simulink library "uavsimBlockset_Environment_turbulentWind"  (Simulink 8.6)
settings: Solver=ode45  StartTime=0.0  StopTime=10.0  RelTol=1e-3
undefined symbols (not defined in the file): F, Light, mask_ambientWind, mask_windON, mask_wingspan, MIL, uavsimblockset_cartesianToAngle
libraries: aerolibwind2 x1
settings Model: Creator=mstolle  LastModifiedBy=j.bolting

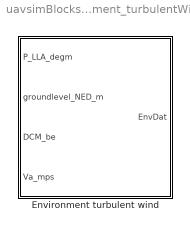
== system uavsimBlockset_Environment_turbulentWind ==
  Environment turbulent wind : Subsystem  mask{mask_constantwind_NED_mps=mask_ambientWind, mask_wingspan=mask_wingspan, mask_windON=mask_windON, mask_turbulenceON=1}
      mask prompts: mask_constantwind_NED_mps "Ambient, i.e. constant wind vector [m/s], NED frame"; mask_wingspan "Aircraft wingspan"; mask_windON "Ambient wind ON?"; mask_turbulenceON "Turbulence ON?"

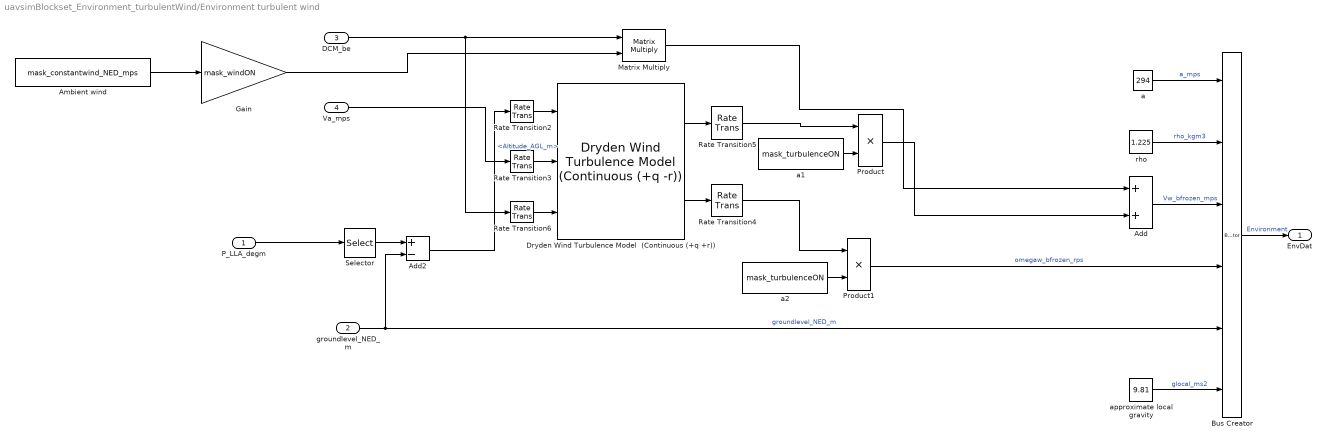
== system uavsimBlockset_Environment_turbulentWind/Environment turbulent wind ==
  P_LLA_degm : Inport
  groundlevel_NED_m : Inport  Port=2
  DCM_be : Inport  Port=3
  Va_mps : Inport  Port=4
  Add : Sum
  Add2 : Sum  Inputs=+-
  Ambient wind : Constant  Value=mask_constantwind_NED_mps
  Bus Creator : BusCreator  Inputs=6  OutDataTypeStr=Bus: Environment  NonVirtualBus=on
  Dryden Wind Turbulence Model  (Continuous (+q +r)) : aerolibwind2/Dryden Wind Turbulence Model  (Continuous (+q -r))  units=Metric (MKS)  spec=MIL-F-8785C  model=Discrete Dryden (+q -r)  W20=norm(mask_constantwind_NED_mps)  Wdeg=rad2deg(uavsimblockset_cartesianToAngle(mask_constantwind_NED_mps(1), mask_constantwind_NED_mps(2)))  TurbProb=10^-2 - Light  L_high=533.4  Wingspan=mask_wingspan  ts=0.1  Seed=randi(2^6, [1 4])  T_on=on
  Gain : Gain  Gain=mask_windON
  Matrix Multiply : Product  Multiplication=Matrix(*)
  Product : Product  RndMeth=Zero
  Product1 : Product  RndMeth=Zero
  Rate Transition2 : RateTransition  OutPortSampleTime=0.1
  Rate Transition3 : RateTransition  OutPortSampleTime=0.1
  Rate Transition4 : RateTransition  OutPortSampleTime=0
  Rate Transition5 : RateTransition  OutPortSampleTime=0
  Rate Transition6 : RateTransition  OutPortSampleTime=0.1
  Selector : Selector  InputPortWidth=3  IndexOptions=Index vector (dialog)  Indices=3  OutputSizes=1
  a : Constant  Value=294
  a1 : Constant  Value=mask_turbulenceON
  a2 : Constant  Value=mask_turbulenceON
  approximate local gravity : Constant  Value=9.81
  "rho " : Constant  Value=1.225
  EnvDat : Outport  OutDataTypeStr=Bus: Environment
  wires:
  Gain/1 -> Matrix Multiply/2
  Product1/1 -> Bus Creator/4  "omegaw_bfrozen_rps"
  a2/1 -> Product1/2
  a1/1 -> Product/2
  Product/1 -> Add/2
  Dryden Wind Turbulence Model  (Continuous (+q +r))/2 -> Rate Transition4/1
  P_LLA_degm/1 -> Selector/1
  groundlevel_NED_m/1 -> Add2/2, Bus Creator/5  "groundlevel_NED_m"
  Bus Creator/1 -> EnvDat/1  "Environment"
  "rho "/1 -> Bus Creator/2  "rho_kgm3"
  a/1 -> Bus Creator/1  "a_mps"
  Add/1 -> Bus Creator/3  "Vw_bfrozen_mps"
  approximate local gravity/1 -> Bus Creator/6  "glocal_ms2"
  Add2/1 -> Rate Transition2/1  "<Altitude_AGL_m>"
  Va_mps/1 -> Rate Transition3/1
  DCM_be/1 -> Matrix Multiply/1, Rate Transition6/1
  Ambient wind/1 -> Gain/1
  Dryden Wind Turbulence Model  (Continuous (+q +r))/1 -> Rate Transition5/1
  Matrix Multiply/1 -> Add/1
  Rate Transition4/1 -> Product1/1
  Rate Transition5/1 -> Product/1
  Selector/1 -> Add2/1
  Rate Transition2/1 -> Dryden Wind Turbulence Model  (Continuous (+q +r))/1
  Rate Transition3/1 -> Dryden Wind Turbulence Model  (Continuous (+q +r))/2
  Rate Transition6/1 -> Dryden Wind Turbulence Model  (Continuous (+q +r))/3
